simulink model "BoostDCDCRegulated"  (Simulink 6.2)
settings: Solver=ode23tb  StartTime=0.0  StopTime=0.1  MaxStep=2e-6  RelTol=1e-3
libraries: powerlib x12, powerlib_extras x1
settings Model: LastModifiedBy=cwang
settings DebuggingCC: SolverPrmCheckMsg=warning

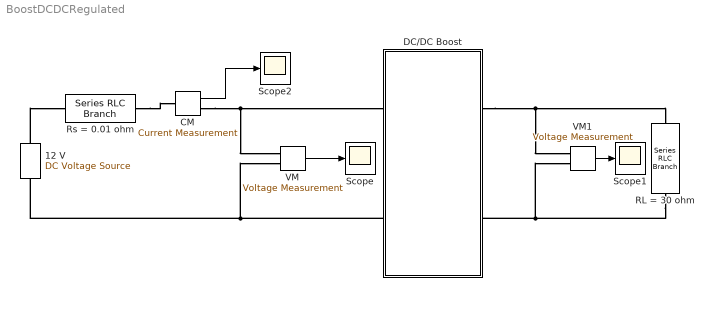
== system BoostDCDCRegulated ==
  12 V : powerlib/Electrical Sources/DC Voltage Source  Orientation=up  Amplitude=12  Measurements=None
  CM : powerlib/Measurements/Current Measurement  PhasorSimulation=off  OutputType=Complex  PSBequivalent=0
  DC/DC Boost : Subsystem
  RL = 30 ohm : powerlib/Elements/Series RLC Branch  Orientation=up  PhysicalDomain=powersysdomain  SubClassName=unknown  LeftPortType=p1  RightPortType=p1  LConnTagsString=__new0  RConnTagsString=__new0  Resistance=50  Inductance=0  Capacitance=inf  Setx0=off  InitialVoltage=0  SetiL0=off  InitialCurrent=0  Measurements=None
  Rs = 0.01 ohm : powerlib/Elements/Series RLC Branch  PhysicalDomain=powersysdomain  SubClassName=unknown  LeftPortType=p1  RightPortType=p1  LConnTagsString=__new0  RConnTagsString=__new0  Resistance=0.01  Inductance=0  Capacitance=inf  Setx0=off  InitialVoltage=0  SetiL0=off  InitialCurrent=0  Measurements=None
  Scope : Scope
      settings: SaveName=Vin
  Scope1 : Scope
      settings: SaveName=Vo
  Scope2 : Scope
      settings: SaveName=IL
  VM : powerlib/Measurements/Voltage Measurement  PhasorSimulation=off  OutputType=Complex  PSBequivalent=0
  VM1 : powerlib/Measurements/Voltage Measurement  PhasorSimulation=off  OutputType=Complex  PSBequivalent=0
  wires:
  VM/1 -> Scope/1
  VM1/1 -> Scope1/1
  CM/1 -> Scope2/1
  connections:
  12 V/RConn1 -- Rs = 0.01 ohm/LConn1
  DC/DC Boost/LConn2 -- 12 V/LConn1 -- VM/LConn2
  DC/DC Boost/RConn1 -- RL = 30 ohm/RConn1 -- VM1/LConn1
  RL = 30 ohm/LConn1 -- DC/DC Boost/RConn2 -- VM1/LConn2
  Rs = 0.01 ohm/RConn1 -- CM/LConn1
  CM/RConn1 -- DC/DC Boost/LConn1 -- VM/LConn1

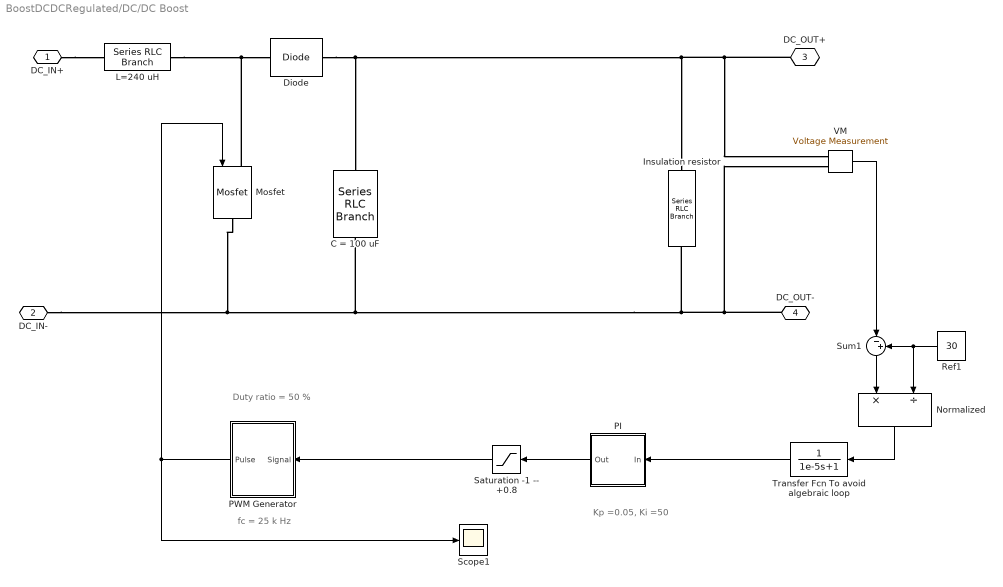
== system BoostDCDCRegulated/DC/DC Boost ==
  note: Duty ratio = 50 %
  note: fc = 25 k Hz
  note: Kp =0.05, Ki =50
  C = 100 uF : powerlib/Elements/Series RLC Branch  Orientation=down  PhysicalDomain=powersysdomain  SubClassName=unknown  LeftPortType=p1  RightPortType=p1  LConnTagsString=__new0  RConnTagsString=__new0  Resistance=0  Inductance=0  Capacitance=100e-6  Setx0=off  InitialVoltage=0  SetiL0=off  InitialCurrent=0  Measurements=Branch current
  Diode : powerlib/Power Electronics/Diode  Ron=0.001  Lon=0  Vf=0.8  IC=0  Rs=500  Cs=250e-9  Measurements=off
  Insulation resistor : powerlib/Elements/Series RLC Branch  Orientation=up  PhysicalDomain=powersysdomain  SubClassName=unknown  LeftPortType=p1  RightPortType=p1  LConnTagsString=__new0  RConnTagsString=__new0  Resistance=1000000  Inductance=0  Capacitance=inf  Setx0=off  InitialVoltage=0  SetiL0=off  InitialCurrent=0  Measurements=Branch voltage
  L=240 uH : powerlib/Elements/Series RLC Branch  PhysicalDomain=powersysdomain  SubClassName=unknown  LeftPortType=p1  RightPortType=p1  LConnTagsString=__new0  RConnTagsString=__new0  Resistance=0  Inductance=240e-6  Capacitance=inf  Setx0=off  InitialVoltage=0  SetiL0=off  InitialCurrent=0  Measurements=None
  Mosfet : powerlib/Power Electronics/Mosfet  Orientation=down  Ron=0.001  Lon=1e-6  Rd=.001  IC=0  Rs=1e5  Cs=inf  Measurements=off
  Normalized : Product  Orientation=down  Inputs=*/  SaturateOnIntegerOverflow=on
  PI : Subsystem  Orientation=left  mask{Kp=0.2, Ki=80, Supper=0.8, Slower=-1, Sini=0}
      mask prompts: Kp "Propotional Gain Kp"; Ki "Integral Gain Ki"; Supper "Integral upper limit"; Slower "Integral lower limit"; Sini "Initial Value of integral"
  PWM Generator : Subsystem  Orientation=left
  Ref1 : Constant  Orientation=left  Value=30
  "Saturation -1 -- +0.8" : Saturate  Orientation=left  UpperLimit=0.8  LowerLimit=-1
  Scope1 : Scope
      settings: SaveName=Vpulse
  Sum1 : Sum  Orientation=down  Inputs=|-+  SaturateOnIntegerOverflow=on
  Transfer Fcn To avoid algebraic loop : TransferFcn  Orientation=left  Denominator=[1e-5 1]
  VM : powerlib/Measurements/Voltage Measurement  PhasorSimulation=off  OutputType=Complex  PSBequivalent=0
  DC_IN+ : PMIOPort  Port=1  Side=Left
  DC_IN- : PMIOPort  Port=2  Side=Left
  DC_OUT+ : PMIOPort  Orientation=left  Port=3  Side=Right
  DC_OUT- : PMIOPort  Orientation=left  Port=4  Side=Right
  wires:
  PWM Generator/1(Pulse) -> Mosfet/1, Scope1/1
  "Saturation -1 -- +0.8"/1 -> PWM Generator/1(Signal)
  PI/1(Out) -> "Saturation -1 -- +0.8"/1
  Transfer Fcn To avoid algebraic loop/1 -> PI/1(In)
  Ref1/1 -> Sum1/2, Normalized/2
  Sum1/1 -> Normalized/1
  Normalized/1 -> Transfer Fcn To avoid algebraic loop/1
  VM/1 -> Sum1/1
  connections:
  Mosfet/LConn1 -- Diode/LConn1 -- L=240 uH/RConn1
  DC_OUT-/RConn1 -- Mosfet/RConn1 -- DC_IN-/RConn1 -- C = 100 uF/RConn1 -- Insulation resistor/LConn1 -- VM/LConn2
  DC_OUT+/RConn1 -- Diode/RConn1 -- C = 100 uF/LConn1 -- Insulation resistor/RConn1 -- VM/LConn1
  DC_IN+/RConn1 -- L=240 uH/LConn1

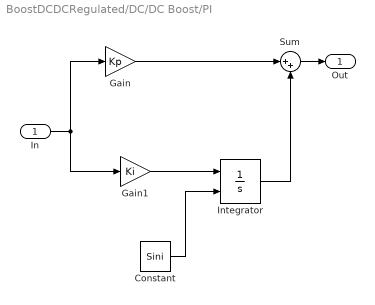
== system BoostDCDCRegulated/DC/DC Boost/PI ==
  In : Inport  Port=1  LatchInput=off
  Constant : Constant  Value=Sini
  Gain : Gain  Gain=Kp  SaturateOnIntegerOverflow=on
  Gain1 : Gain  Gain=Ki  SaturateOnIntegerOverflow=on
  Integrator : Integrator  InitialConditionSource=external  LimitOutput=on  UpperSaturationLimit=Supper  LowerSaturationLimit=Slower
  Sum : Sum  Inputs=|++  SaturateOnIntegerOverflow=on
  Out : Outport
  wires:
  Constant/1 -> Integrator/2
  Gain/1 -> Sum/1
  In/1 -> Gain1/1, Gain/1
  Gain1/1 -> Integrator/1
  Integrator/1 -> Sum/2
  Sum/1 -> Out/1

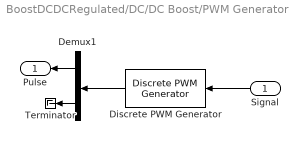
== system BoostDCDCRegulated/DC/DC Boost/PWM Generator ==
  Signal : Inport  Orientation=left  Port=1  LatchInput=off
  Demux1 : Demux  Orientation=left  Outputs=2
  Discrete PWM Generator : powerlib_extras/Discrete  Control Blocks/Discrete PWM Generator  Orientation=left  GeneratorMode="1-arm  bridge (2 pulses)"  Fc=25e3  Ts=4e-6  Internal=off  mIndex=0.4  Freq=60  Phase=0
  Terminator : Terminator
  Pulse : Outport  Orientation=left
  wires:
  Discrete PWM Generator/1 -> Demux1/1
  Signal/1 -> Discrete PWM Generator/1
  Demux1/1 -> Pulse/1
  Demux1/2 -> Terminator/1
